simulink library "MBDS_Applications"  (R2018b)
settings: Solver=ode45  StartTime=0.0  StopTime=10.0  RelTol=1e-3
undefined symbols (not defined in the file or in its folder): Ts
libraries: KIBES_Signal x297, simulink x7
(part 2 of 6)

== system MBDS_Applications/APP_MyApplication/DM1TX ==
  note: DM1TX
  Constant6 : Constant  InitFcn=|  OutDataTypeStr=boolean
      | if(exist('MBDS_BlockCallback', 'file'))
      |    MBDS_BlockCallback('Update', gcb);  
      | end
  Constant8 : Constant  InitFcn=|  Value=0  OutDataTypeStr=boolean
      | if(exist('MBDS_BlockCallback', 'file'))
      |    MBDS_BlockCallback('Update', gcb);  
      | end
  Switch : Switch  InitFcn=|  Criteria=u2 ~= 0  OutDataTypeStr=Inherit: Inherit via back propagation  mask(Switch){MBDS_LibraryBlock=on, OutDataTypeStr_=Inherit: Inherit via back propagation, SaturateOnIntegerOverflow_=off, InputSameDT_=off, MBDS_BlockVersion=07.21.05}
      | if(exist('MBDS_BlockCallback', 'file'))
      |    MBDS_BlockCallback('Update', gcb);  
      | end
      mask prompts: MBDS_LibraryBlock "MBDS library block"; OutDataTypeStr_ "Output data type:"; SaturateOnIntegerOverflow_ "Saturate on integer overflow"; InputSameDT_ "Require all inputs to have the same data type"; MBDS_BlockVersion "Block version:"
      mask help: Pass through input 1 when input 2 is not equal to zero; otherwise pass through input 3. The inputs are numbered top to bottom (or left to right). The first and third input ports are data ports, and the second input port is the control port.
      mask init: same as MBDS_Applications/APP_MyApplication/NOT
      mask Help: eval(['open([workdir(''library_dir:''),''\Blockset\help\'',get_param(gcb,''MaskType''),''.html''])'])
      mask TypeOptions OutDataTypeStr_: Inherit: Inherit via back propagation | single | int8 | uint8 | int16 | uint16 | int32 | uint32
      mask DialogControl ParameterTabVar0 Prompt: Signal Attributes
      mask DialogControl ParameterTabVar01 Prompt: Version
  in_DCAN.GenericDM1TxMessage.DeviceState : KIBES_Signal/KIBES_Signal  MBDS_LibraryBlock=on  DatabaseKey=202  SignalName=DCAN.GenericDM1TxMessage.DeviceState  SymbolName=DCAN_GenericDM1TxMessage_DeviceState_000202  DataType=uint16  Init=0  Slope=1  Bias=0  DataSize=1  fpDataType=uint16  BlockIOType=Inport  DeviceType=0
  in_FMSCAN.GenericDM1TxMessage.DeviceState : KIBES_Signal/KIBES_Signal  MBDS_LibraryBlock=on  DatabaseKey=340  SignalName=FMSCAN.GenericDM1TxMessage.DeviceState  SymbolName=FMSCAN_GenericDM1TxMessage_DeviceState_000340  DataType=uint16  Init=0  Slope=1  Bias=0  DataSize=1  fpDataType=uint16  BlockIOType=Inport  DeviceType=0
  in_PCAN.GenericDM1TxMessage.DeviceState : KIBES_Signal/KIBES_Signal  MBDS_LibraryBlock=on  DatabaseKey=338  SignalName=PCAN.GenericDM1TxMessage.DeviceState  SymbolName=PCAN_GenericDM1TxMessage_DeviceState_000338  DataType=uint16  Init=0  Slope=1  Bias=0  DataSize=1  fpDataType=uint16  BlockIOType=Inport  DeviceType=0
  in_STIMD.DTC_enable : KIBES_Signal/KIBES_Signal  MBDS_LibraryBlock=on  DatabaseKey=200  SignalName=STIMD.DTC_enable  SymbolName=STIMD_DTC_enable_000200  DataType=boolean  Init=0  Slope=1  Bias=0  DataSize=1  fpDataType=boolean  BlockIOType=Inport  DeviceType=2
  out_DCAN.GenericDM1TxMessage.DeviceEnable : KIBES_Signal/KIBES_Signal  MBDS_LibraryBlock=on  DatabaseKey=201  SignalName=DCAN.GenericDM1TxMessage.DeviceEnable  SymbolName=DCAN_GenericDM1TxMessage_DeviceEnable_000201  DataType=boolean  Init=0  Slope=1  Bias=0  DataSize=1  fpDataType=boolean  BlockIOType=Outport  DeviceType=0
  out_FMSCAN.GenericDM1TxMessage.DeviceEnable : KIBES_Signal/KIBES_Signal  MBDS_LibraryBlock=on  DatabaseKey=341  SignalName=FMSCAN.GenericDM1TxMessage.DeviceEnable  SymbolName=FMSCAN_GenericDM1TxMessage_DeviceEnable_000341  DataType=boolean  Init=0  Slope=1  Bias=0  DataSize=1  fpDataType=boolean  BlockIOType=Outport  DeviceType=0
  out_PCAN.GenericDM1TxMessage.DeviceEnable : KIBES_Signal/KIBES_Signal  MBDS_LibraryBlock=on  DatabaseKey=339  SignalName=PCAN.GenericDM1TxMessage.DeviceEnable  SymbolName=PCAN_GenericDM1TxMessage_DeviceEnable_000339  DataType=boolean  Init=0  Slope=1  Bias=0  DataSize=1  fpDataType=boolean  BlockIOType=Outport  DeviceType=0
  wires:
  in_STIMD.DTC_enable/1 -> Switch/2
  Constant6/1 -> Switch/1
  Constant8/1 -> Switch/3
  Switch/1 -> out_FMSCAN.GenericDM1TxMessage.DeviceEnable/1, out_PCAN.GenericDM1TxMessage.DeviceEnable/1, out_DCAN.GenericDM1TxMessage.DeviceEnable/1

== system MBDS_Applications/APP_MyApplication/DM2_3_11 ==
  Constant1 : Constant  InitFcn=|  OutDataTypeStr=boolean
      | if(exist('MBDS_BlockCallback', 'file'))
      |    MBDS_BlockCallback('Update', gcb);  
      | end
  Constant2 : Constant  InitFcn=|  OutDataTypeStr=boolean
      | if(exist('MBDS_BlockCallback', 'file'))
      |    MBDS_BlockCallback('Update', gcb);  
      | end
  Constant3 : Constant  InitFcn=|  OutDataTypeStr=boolean
      | if(exist('MBDS_BlockCallback', 'file'))
      |    MBDS_BlockCallback('Update', gcb);  
      | end
  OR1 : Subsystem  InitFcn=|  mask(OR){MBDS_LibraryBlock=on, BitwiseMode=off, Inputs=2, UseBitMask=off, BitMask='A1', OutDataTypeStr=Inherit: Inherit via back propagation, MBDS_BlockVersion=07.21.05}
      | if(exist('MBDS_BlockCallback', 'file'))
      |    MBDS_BlockCallback('Update', gcb);
      | end
      mask prompts: MBDS_LibraryBlock "MBDS library block"; BitwiseMode "Use 'bitwise' mode"; Inputs "Number of input ports:"; UseBitMask "Use bit mask"; BitMask "Bit mask:"; OutDataTypeStr "Output data type:"; MBDS_BlockVersion "Version:"
      mask help: Logical or bitwise OR operator. For multiple inputs, operators are applied across the inputs. For a single input, operators are applied across the input vector. In bitwise mode a bit mask can be applied onto single input signals.
      mask init: same as MBDS_Applications/APP_MyApplication/NOT
      mask Help: eval(['open([workdir(''library_dir:''),''\Blockset\help\'',get_param(gcb,''MaskType''),''.html''])'])
      mask Callback BitwiseMode:
      | if(exist('MBDS_BlockCallback', 'file'))
      |    MBDS_BlockCallback('BitwiseMode', gcb);
      | end
      mask Callback Inputs:
      | if(exist('MBDS_BlockCallback', 'file'))
      |    MBDS_BlockCallback('Inputs', gcb);
      | end
      mask Callback UseBitMask:
      | if(exist('MBDS_BlockCallback', 'file'))
      |    MBDS_BlockCallback('UseBitMask', gcb);
      | end
      mask Callback BitMask:
      | if(exist('MBDS_BlockCallback', 'file'))
      |    MBDS_BlockCallback('BitMask', gcb);
      | end
      mask TypeOptions OutDataTypeStr: Inherit: Inherit via back propagation | int8 | uint8 | int16 | uint16 | int32 | uint32 | boolean
      mask Callback OutDataTypeStr:
      | % Adopt Value
      | if(exist('MBDS_BlockCallback', 'file'))
      |    MBDS_BlockCallback('OutDataTypeStr', gcb);
      | end
      mask DialogControl ParameterTabVar0 Prompt: Main
      mask DialogControl ParameterTabVar01 Prompt: Signal Attributes
      mask DialogControl ParameterTabVar012 Prompt: Version
      mask Display:
      | % Show icon or block text
      | if(UseBitMask)
      |    if(isnumeric(BitMask))
      |       BitMaskString = ['0x',dec2hex(floor(BitMask))];
      |    elseif(ischar(BitMask))
      |       BitMaskString = ['0x',upper(BitMask)];
      |    else
      |       BitMaskString = '???';
      |    end
      |    disp(sprintf(['OR\n', BitMaskString]))
      | else
      |    disp('OR')
      | end
  OR2 : Subsystem  InitFcn=|  mask(OR){MBDS_LibraryBlock=on, BitwiseMode=off, Inputs=2, UseBitMask=off, BitMask='A1', OutDataTypeStr=Inherit: Inherit via back propagation, MBDS_BlockVersion=07.21.05}
      | if(exist('MBDS_BlockCallback', 'file'))
      |    MBDS_BlockCallback('Update', gcb);
      | end
      mask prompts: MBDS_LibraryBlock "MBDS library block"; BitwiseMode "Use 'bitwise' mode"; Inputs "Number of input ports:"; UseBitMask "Use bit mask"; BitMask "Bit mask:"; OutDataTypeStr "Output data type:"; MBDS_BlockVersion "Version:"
      mask help: Logical or bitwise OR operator. For multiple inputs, operators are applied across the inputs. For a single input, operators are applied across the input vector. In bitwise mode a bit mask can be applied onto single input signals.
      mask init: same as MBDS_Applications/APP_MyApplication/NOT
      mask Help: eval(['open([workdir(''library_dir:''),''\Blockset\help\'',get_param(gcb,''MaskType''),''.html''])'])
      mask Callback BitwiseMode:
      | if(exist('MBDS_BlockCallback', 'file'))
      |    MBDS_BlockCallback('BitwiseMode', gcb);
      | end
      mask Callback Inputs:
      | if(exist('MBDS_BlockCallback', 'file'))
      |    MBDS_BlockCallback('Inputs', gcb);
      | end
      mask Callback UseBitMask:
      | if(exist('MBDS_BlockCallback', 'file'))
      |    MBDS_BlockCallback('UseBitMask', gcb);
      | end
      mask Callback BitMask:
      | if(exist('MBDS_BlockCallback', 'file'))
      |    MBDS_BlockCallback('BitMask', gcb);
      | end
      mask TypeOptions OutDataTypeStr: Inherit: Inherit via back propagation | int8 | uint8 | int16 | uint16 | int32 | uint32 | boolean
      mask Callback OutDataTypeStr:
      | % Adopt Value
      | if(exist('MBDS_BlockCallback', 'file'))
      |    MBDS_BlockCallback('OutDataTypeStr', gcb);
      | end
      mask DialogControl ParameterTabVar0 Prompt: Main
      mask DialogControl ParameterTabVar01 Prompt: Signal Attributes
      mask DialogControl ParameterTabVar012 Prompt: Version
      mask Display:
      | % Show icon or block text
      | if(UseBitMask)
      |    if(isnumeric(BitMask))
      |       BitMaskString = ['0x',dec2hex(floor(BitMask))];
      |    elseif(ischar(BitMask))
      |       BitMaskString = ['0x',upper(BitMask)];
      |    else
      |       BitMaskString = '???';
      |    end
      |    disp(sprintf(['OR\n', BitMaskString]))
      | else
      |    disp('OR')
      | end
  OR3 : Subsystem  InitFcn=|  mask(OR){MBDS_LibraryBlock=on, BitwiseMode=off, Inputs=2, UseBitMask=off, BitMask='A1', OutDataTypeStr=Inherit: Inherit via back propagation, MBDS_BlockVersion=07.21.05}
      | if(exist('MBDS_BlockCallback', 'file'))
      |    MBDS_BlockCallback('Update', gcb);
      | end
      mask prompts: MBDS_LibraryBlock "MBDS library block"; BitwiseMode "Use 'bitwise' mode"; Inputs "Number of input ports:"; UseBitMask "Use bit mask"; BitMask "Bit mask:"; OutDataTypeStr "Output data type:"; MBDS_BlockVersion "Version:"
      mask help: Logical or bitwise OR operator. For multiple inputs, operators are applied across the inputs. For a single input, operators are applied across the input vector. In bitwise mode a bit mask can be applied onto single input signals.
      mask init: same as MBDS_Applications/APP_MyApplication/NOT
      mask Help: eval(['open([workdir(''library_dir:''),''\Blockset\help\'',get_param(gcb,''MaskType''),''.html''])'])
      mask Callback BitwiseMode:
      | if(exist('MBDS_BlockCallback', 'file'))
      |    MBDS_BlockCallback('BitwiseMode', gcb);
      | end
      mask Callback Inputs:
      | if(exist('MBDS_BlockCallback', 'file'))
      |    MBDS_BlockCallback('Inputs', gcb);
      | end
      mask Callback UseBitMask:
      | if(exist('MBDS_BlockCallback', 'file'))
      |    MBDS_BlockCallback('UseBitMask', gcb);
      | end
      mask Callback BitMask:
      | if(exist('MBDS_BlockCallback', 'file'))
      |    MBDS_BlockCallback('BitMask', gcb);
      | end
      mask TypeOptions OutDataTypeStr: Inherit: Inherit via back propagation | int8 | uint8 | int16 | uint16 | int32 | uint32 | boolean
      mask Callback OutDataTypeStr:
      | % Adopt Value
      | if(exist('MBDS_BlockCallback', 'file'))
      |    MBDS_BlockCallback('OutDataTypeStr', gcb);
      | end
      mask DialogControl ParameterTabVar0 Prompt: Main
      mask DialogControl ParameterTabVar01 Prompt: Signal Attributes
      mask DialogControl ParameterTabVar012 Prompt: Version
      mask Display:
      | % Show icon or block text
      | if(UseBitMask)
      |    if(isnumeric(BitMask))
      |       BitMaskString = ['0x',dec2hex(floor(BitMask))];
      |    elseif(ischar(BitMask))
      |       BitMaskString = ['0x',upper(BitMask)];
      |    else
      |       BitMaskString = '???';
      |    end
      |    disp(sprintf(['OR\n', BitMaskString]))
      | else
      |    disp('OR')
      | end
  in_DCAN.GenericDM11RXMessage.DeviceState : KIBES_Signal/KIBES_Signal  MBDS_LibraryBlock=on  DatabaseKey=396  SignalName=DCAN.GenericDM11RXMessage.DeviceState  SymbolName=DCAN_GenericDM11RXMessage_DeviceState_000396  DataType=uint16  Init=0  Slope=1  Bias=0  DataSize=1  fpDataType=uint16  BlockIOType=Inport  DeviceType=0
  in_DCAN.GenericDM2TxMessage.Device_State : KIBES_Signal/KIBES_Signal  MBDS_LibraryBlock=on  DatabaseKey=392  SignalName=DCAN.GenericDM2TxMessage.Device_State  SymbolName=DCAN_GenericDM2TxMessage_Device_State_000392  DataType=uint16  Init=0  Slope=1  Bias=0  DataSize=1  fpDataType=uint16  BlockIOType=Inport  DeviceType=0
  in_DCAN.GenericDM3RxMessage.Device_State : KIBES_Signal/KIBES_Signal  MBDS_LibraryBlock=on  DatabaseKey=394  SignalName=DCAN.GenericDM3RxMessage.Device_State  SymbolName=DCAN_GenericDM3RxMessage_Device_State_000394  DataType=uint16  Init=0  Slope=1  Bias=0  DataSize=1  fpDataType=uint16  BlockIOType=Inport  DeviceType=0
  in_STIMD.DM11_enable : KIBES_Signal/KIBES_Signal  MBDS_LibraryBlock=on  DatabaseKey=398  SignalName=STIMD.DM11_enable  SymbolName=STIMD_DM11_enable_000398  DataType=boolean  Init=0  Slope=1  Bias=0  DataSize=1  fpDataType=boolean  BlockIOType=Inport  DeviceType=2
  in_STIMD.DM2_enable : KIBES_Signal/KIBES_Signal  MBDS_LibraryBlock=on  DatabaseKey=399  SignalName=STIMD.DM2_enable  SymbolName=STIMD_DM2_enable_000399  DataType=boolean  Init=0  Slope=1  Bias=0  DataSize=1  fpDataType=boolean  BlockIOType=Inport  DeviceType=2
  in_STIMD.DM3_enable : KIBES_Signal/KIBES_Signal  MBDS_LibraryBlock=on  DatabaseKey=400  SignalName=STIMD.DM3_enable  SymbolName=STIMD_DM3_enable_000400  DataType=boolean  Init=0  Slope=1  Bias=0  DataSize=1  fpDataType=boolean  BlockIOType=Inport  DeviceType=2
  out_DCAN.GenericDM11RXMessage.DeviceEnable : KIBES_Signal/KIBES_Signal  MBDS_LibraryBlock=on  DatabaseKey=397  SignalName=DCAN.GenericDM11RXMessage.DeviceEnable  SymbolName=DCAN_GenericDM11RXMessage_DeviceEnable_000397  DataType=boolean  Init=0  Slope=1  Bias=0  DataSize=1  fpDataType=boolean  BlockIOType=Outport  DeviceType=0
  out_DCAN.GenericDM2TxMessage.Device_Enable : KIBES_Signal/KIBES_Signal  MBDS_LibraryBlock=on  DatabaseKey=393  SignalName=DCAN.GenericDM2TxMessage.Device_Enable  SymbolName=DCAN_GenericDM2TxMessage_Device_Enable_000393  DataType=boolean  Init=0  Slope=1  Bias=0  DataSize=1  fpDataType=boolean  BlockIOType=Outport  DeviceType=0
  out_DCAN.GenericDM3RxMessage.Device_Enable : KIBES_Signal/KIBES_Signal  MBDS_LibraryBlock=on  DatabaseKey=395  SignalName=DCAN.GenericDM3RxMessage.Device_Enable  SymbolName=DCAN_GenericDM3RxMessage_Device_Enable_000395  DataType=boolean  Init=0  Slope=1  Bias=0  DataSize=1  fpDataType=boolean  BlockIOType=Outport  DeviceType=0
  wires:
  in_STIMD.DM3_enable/1 -> OR3/1(u1)
  OR3/1(y) -> out_DCAN.GenericDM3RxMessage.Device_Enable/1
  Constant3/1 -> OR3/2(u2)
  in_STIMD.DM2_enable/1 -> OR2/1(u1)
  OR2/1(y) -> out_DCAN.GenericDM2TxMessage.Device_Enable/1
  Constant2/1 -> OR2/2(u2)
  in_STIMD.DM11_enable/1 -> OR1/1(u1)
  OR1/1(y) -> out_DCAN.GenericDM11RXMessage.DeviceEnable/1
  Constant1/1 -> OR1/2(u2)

== system MBDS_Applications/APP_MyApplication/DM4RX ==
  note: F1 = 241
  Constant1 : Constant  InitFcn=|  OutDataTypeStr=boolean
      | if(exist('MBDS_BlockCallback', 'file'))
      |    MBDS_BlockCallback('Update', gcb);  
      | end
  Constant2 : Constant  InitFcn=|  OutDataTypeStr=boolean
      | if(exist('MBDS_BlockCallback', 'file'))
      |    MBDS_BlockCallback('Update', gcb);  
      | end
  in_DM4RXMainDevice.FaultIndication : KIBES_Signal/KIBES_Signal  MBDS_LibraryBlock=on  DatabaseKey=322  SignalName=DM4RXMainDevice.FaultIndication  SymbolName=DM4RXMainDevice_FaultIndication_000322  DataType=boolean  Init=0  Slope=1  Bias=0  DataSize=1  fpDataType=boolean  BlockIOType=Inport  DeviceType=0
  in_DM4RXMainDevice.FirstEntry : KIBES_Signal/KIBES_Signal  MBDS_LibraryBlock=on  DatabaseKey=323  SignalName=DM4RXMainDevice.FirstEntry  SymbolName=DM4RXMainDevice_FirstEntry_000323  DataType=boolean  Init=0  Slope=1  Bias=0  DataSize=1  fpDataType=boolean  BlockIOType=Inport  DeviceType=0
  in_DM4RXMainDevice.Fmi : KIBES_Signal/KIBES_Signal  MBDS_LibraryBlock=on  DatabaseKey=324  SignalName=DM4RXMainDevice.Fmi  SymbolName=DM4RXMainDevice_Fmi_000324  DataType=uint8  Init=0  Slope=1  Bias=0  DataSize=1  fpDataType=uint8  BlockIOType=Inport  DeviceType=0
  in_DM4RXMainDevice.LastEntry : KIBES_Signal/KIBES_Signal  MBDS_LibraryBlock=on  DatabaseKey=325  SignalName=DM4RXMainDevice.LastEntry  SymbolName=DM4RXMainDevice_LastEntry_000325  DataType=boolean  Init=0  Slope=1  Bias=0  DataSize=1  fpDataType=boolean  BlockIOType=Inport  DeviceType=0
  in_DM4RXMainDevice.NumberOfDtcs : KIBES_Signal/KIBES_Signal  MBDS_LibraryBlock=on  DatabaseKey=327  SignalName=DM4RXMainDevice.NumberOfDtcs  SymbolName=DM4RXMainDevice_NumberOfDtcs_000327  DataType=uint8  Init=0  Slope=1  Bias=0  DataSize=1  fpDataType=uint8  BlockIOType=Inport  DeviceType=0
  in_DM4RXMainDevice.OccCount : KIBES_Signal/KIBES_Signal  MBDS_LibraryBlock=on  DatabaseKey=328  SignalName=DM4RXMainDevice.OccCount  SymbolName=DM4RXMainDevice_OccCount_000328  DataType=uint8  Init=0  Slope=1  Bias=0  DataSize=1  fpDataType=uint8  BlockIOType=Inport  DeviceType=0
  in_DM4RXMainDevice.Spn : KIBES_Signal/KIBES_Signal  MBDS_LibraryBlock=on  DatabaseKey=331  SignalName=DM4RXMainDevice.Spn  SymbolName=DM4RXMainDevice_Spn_000331  DataType=uint32  Init=0  Slope=1  Bias=0  DataSize=1  fpDataType=uint32  BlockIOType=Inport  DeviceType=0
  in_PCAN.GenericDM4REQ.DeviceState : KIBES_Signal/KIBES_Signal  MBDS_LibraryBlock=on  DatabaseKey=319  SignalName=PCAN.GenericDM4REQ.DeviceState  SymbolName=PCAN_GenericDM4REQ_DeviceState_000319  DataType=uint16  Init=0  Slope=1  Bias=0  DataSize=1  fpDataType=uint16  BlockIOType=Inport  DeviceType=0
  in_STIMD.DM4RX_EcuAddress : KIBES_Signal/KIBES_Signal  MBDS_LibraryBlock=on  DatabaseKey=333  SignalName=STIMD.DM4RX_EcuAddress  SymbolName=STIMD_DM4RX_EcuAddress_000333  DataType=uint8  Init=241  Slope=1  Bias=0  DataSize=1  fpDataType=uint8  BlockIOType=Inport  DeviceType=2
  in_STIMD.DM4RX_Next : KIBES_Signal/KIBES_Signal  MBDS_LibraryBlock=on  DatabaseKey=334  SignalName=STIMD.DM4RX_Next  SymbolName=STIMD_DM4RX_Next_000334  DataType=boolean  Init=0  Slope=1  Bias=0  DataSize=1  fpDataType=boolean  BlockIOType=Inport  DeviceType=2
  in_STIMD.DM4RX_Previous : KIBES_Signal/KIBES_Signal  MBDS_LibraryBlock=on  DatabaseKey=332  SignalName=STIMD.DM4RX_Previous  SymbolName=STIMD_DM4RX_Previous_000332  DataType=boolean  Init=0  Slope=1  Bias=0  DataSize=1  fpDataType=boolean  BlockIOType=Inport  DeviceType=2
  in_STIMD.DM4RX_RequestDm4 : KIBES_Signal/KIBES_Signal  MBDS_LibraryBlock=on  DatabaseKey=335  SignalName=STIMD.DM4RX_RequestDm4  SymbolName=STIMD_DM4RX_RequestDm4_000335  DataType=boolean  Init=0  Slope=1  Bias=0  DataSize=1  fpDataType=boolean  BlockIOType=Inport  DeviceType=2
  out_DM4RXMainDevice.EcuAddress : KIBES_Signal/KIBES_Signal  MBDS_LibraryBlock=on  DatabaseKey=321  SignalName=DM4RXMainDevice.EcuAddress  SymbolName=DM4RXMainDevice_EcuAddress_000321  DataType=uint8  Init=0  Slope=1  Bias=0  DataSize=1  fpDataType=uint8  BlockIOType=Outport  DeviceType=0
  out_DM4RXMainDevice.NextEntry : KIBES_Signal/KIBES_Signal  MBDS_LibraryBlock=on  DatabaseKey=326  SignalName=DM4RXMainDevice.NextEntry  SymbolName=DM4RXMainDevice_NextEntry_000326  DataType=boolean  Init=0  Slope=1  Bias=0  DataSize=1  fpDataType=boolean  BlockIOType=Outport  DeviceType=0
  out_DM4RXMainDevice.PreviousEntry : KIBES_Signal/KIBES_Signal  MBDS_LibraryBlock=on  DatabaseKey=329  SignalName=DM4RXMainDevice.PreviousEntry  SymbolName=DM4RXMainDevice_PreviousEntry_000329  DataType=boolean  Init=0  Slope=1  Bias=0  DataSize=1  fpDataType=boolean  BlockIOType=Outport  DeviceType=0
  out_DM4RXMainDevice.SAEJ1939Format : KIBES_Signal/KIBES_Signal  MBDS_LibraryBlock=on  DatabaseKey=330  SignalName=DM4RXMainDevice.SAEJ1939Format  SymbolName=DM4RXMainDevice_SAEJ1939Format_000330  DataType=boolean  Init=0  Slope=1  Bias=0  DataSize=1  fpDataType=boolean  BlockIOType=Outport  DeviceType=0
  out_PCAN.GenericDM4REQ.DeviceEnable : KIBES_Signal/KIBES_Signal  MBDS_LibraryBlock=on  DatabaseKey=318  SignalName=PCAN.GenericDM4REQ.DeviceEnable  SymbolName=PCAN_GenericDM4REQ_DeviceEnable_000318  DataType=boolean  Init=0  Slope=1  Bias=0  DataSize=1  fpDataType=boolean  BlockIOType=Outport  DeviceType=0
  out_PCAN.GenericDM4REQ.RequestDM4 : KIBES_Signal/KIBES_Signal  MBDS_LibraryBlock=on  DatabaseKey=320  SignalName=PCAN.GenericDM4REQ.RequestDM4  SymbolName=PCAN_GenericDM4REQ_RequestDM4_000320  DataType=boolean  Init=0  Slope=1  Bias=0  DataSize=1  fpDataType=boolean  BlockIOType=Outport  DeviceType=0
  wires:
  in_STIMD.DM4RX_RequestDm4/1 -> out_PCAN.GenericDM4REQ.RequestDM4/1
  Constant2/1 -> out_PCAN.GenericDM4REQ.DeviceEnable/1
  in_STIMD.DM4RX_EcuAddress/1 -> out_DM4RXMainDevice.EcuAddress/1
  in_STIMD.DM4RX_Previous/1 -> out_DM4RXMainDevice.PreviousEntry/1
  in_STIMD.DM4RX_Next/1 -> out_DM4RXMainDevice.NextEntry/1
  Constant1/1 -> out_DM4RXMainDevice.SAEJ1939Format/1

== system MBDS_Applications/APP_MyApplication/DR-CAN ==
  note: 18010621
  Constant1 : Constant  InitFcn=|  Value=66  OutDataTypeStr=uint8
      | if(exist('MBDS_BlockCallback', 'file'))
      |    MBDS_BlockCallback('Update', gcb);  
      | end
  Constant3 : Constant  InitFcn=|  OutDataTypeStr=boolean
      | if(exist('MBDS_BlockCallback', 'file'))
      |    MBDS_BlockCallback('Update', gcb);  
      | end
  in_DRCAN.TX_GEN.DRGenTX_1.MessageState : KIBES_Signal/KIBES_Signal  MBDS_LibraryBlock=on  DatabaseKey=301  SignalName=DRCAN.TX_GEN.DRGenTX_1.MessageState  SymbolName=DRCAN_TX_GEN_DRGenTX_1_MessageState_000301  DataType=uint16  Init=0  Slope=1  Bias=0  DataSize=1  fpDataType=uint16  BlockIOType=Inport  DeviceType=0
  out_DRCAN.TX_GEN.DRGenTX_1.MessageEnable : KIBES_Signal/KIBES_Signal  MBDS_LibraryBlock=on  DatabaseKey=300  SignalName=DRCAN.TX_GEN.DRGenTX_1.MessageEnable  SymbolName=DRCAN_TX_GEN_DRGenTX_1_MessageEnable_000300  DataType=boolean  Init=0  Slope=1  Bias=0  DataSize=1  fpDataType=boolean  BlockIOType=Outport  DeviceType=0
  out_DRCAN.TX_GEN.DRGenTX_1.Val_1 : KIBES_Signal/KIBES_Signal  MBDS_LibraryBlock=on  DatabaseKey=302  SignalName=DRCAN.TX_GEN.DRGenTX_1.Val_1  SymbolName=DRCAN_TX_GEN_DRGenTX_1_Val_1_000302  DataType=uint8  Init=0  Slope=1  Bias=0  DataSize=1  fpDataType=uint8  BlockIOType=Outport  DeviceType=0
  wires:
  Constant1/1 -> out_DRCAN.TX_GEN.DRGenTX_1.Val_1/1
  Constant3/1 -> out_DRCAN.TX_GEN.DRGenTX_1.MessageEnable/1
